simulink model "Nparticles"  (R2025b)
settings: Solver=ode45  StartTime=0.0  StopTime=T  MaxStep=.1  RelTol=1e-5  AbsTol=1e-6
values from neighbouring files (symbols this model uses):
  k = [1, 1, 2, .5]    [bertrand_simulation_Nagents.m]
  q0 = [0; 0; pi/4; 1; 0; pi]    [bertrand_simulation_2agent.m]    (also in bertrand_simulation_Nagents.m = [0, 0, 0,     0, .5, 0,     0, 1, 0,     0, 1.5, 0,     0, 2)
settings Model: Creator=xincheng  LastModifiedBy=xincheng

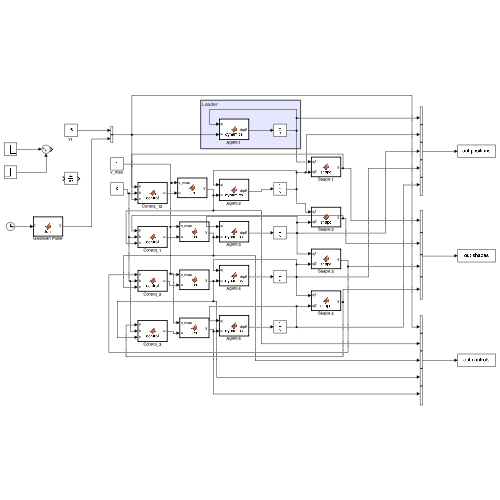
[thumbnail: Simulink's stored preview of the top-level diagram]
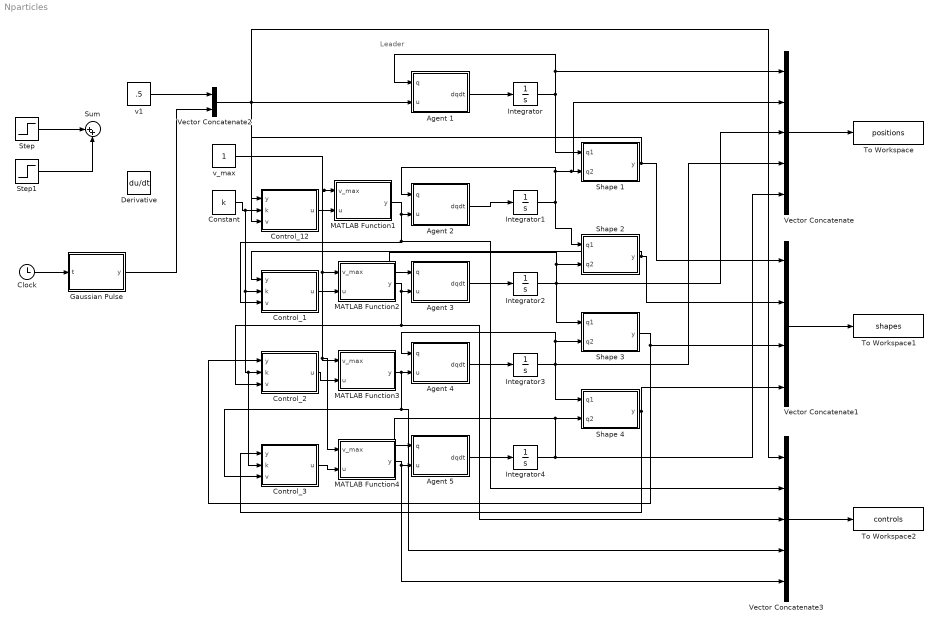
== system Nparticles ==
  note: Leader
  Agent 1 : MATLAB Function  TreatAsAtomicUnit=on
  Agent 2 : MATLAB Function  TreatAsAtomicUnit=on
  Agent 3 : MATLAB Function  TreatAsAtomicUnit=on
  Agent 4 : MATLAB Function  TreatAsAtomicUnit=on
  Agent 5 : MATLAB Function  TreatAsAtomicUnit=on
  Clock : Clock
  Constant : Constant  Value=k
  Control_1 : MATLAB Function  TreatAsAtomicUnit=on
  Control_12 : MATLAB Function  TreatAsAtomicUnit=on
  Control_2 : MATLAB Function  TreatAsAtomicUnit=on
  Control_3 : MATLAB Function  TreatAsAtomicUnit=on
  Derivative : Derivative
  Gaussian Pulse : MATLAB Function  TreatAsAtomicUnit=on
  Integrator : Integrator  InitialCondition=q0(1:3)
  Integrator1 : Integrator  InitialCondition=q0(4:6)
  Integrator2 : Integrator  InitialCondition=q0(7:9)
  Integrator3 : Integrator  InitialCondition=q0(10:12)
  Integrator4 : Integrator  InitialCondition=q0(13:15)
  MATLAB Function1 : MATLAB Function  TreatAsAtomicUnit=on
  MATLAB Function2 : MATLAB Function  TreatAsAtomicUnit=on
  MATLAB Function3 : MATLAB Function  TreatAsAtomicUnit=on
  MATLAB Function4 : MATLAB Function  TreatAsAtomicUnit=on
  Shape 1 : MATLAB Function  TreatAsAtomicUnit=on
  Shape 2 : MATLAB Function  TreatAsAtomicUnit=on
  Shape 3 : MATLAB Function  TreatAsAtomicUnit=on
  Shape 4 : MATLAB Function  TreatAsAtomicUnit=on
  Step : Step  Time=10  After=-2  SampleTime=0
  Step1 : Step  Time=11  After=2  SampleTime=0
  Sum : Sum  Inputs=|++
  To Workspace : ToWorkspace  VariableName=positions  SaveFormat=Timeseries  SampleTime=-1
  To Workspace1 : ToWorkspace  VariableName=shapes  SaveFormat=Timeseries  SampleTime=-1
  To Workspace2 : ToWorkspace  VariableName=controls  SaveFormat=Timeseries  SampleTime=-1
  Vector Concatenate : Concatenate  NumInputs=5
  Vector Concatenate1 : Concatenate  NumInputs=4
  Vector Concatenate2 : Concatenate
  Vector Concatenate3 : Concatenate  NumInputs=5
  v1 : Constant  Value=.5
  v_max : Constant
  wires:
  Agent 1/1(dqdt) -> Integrator/1
  Integrator/1 -> Shape 1/1(q1), Vector Concatenate/1, Agent 1/1(q)
  Integrator1/1 -> Shape 2/1(q1), Agent 2/1(q), Vector Concatenate/2, Shape 1/2(q2)
  Agent 2/1(dqdt) -> Integrator1/1
  Agent 3/1(dqdt) -> Integrator2/1
  Shape 1/1(y) -> Vector Concatenate1/1, Control_12/1(y)
  Control_12/1(u) -> MATLAB Function1/2(u)
  Shape 2/1(y) -> Control_1/1(y), Vector Concatenate1/2
  Control_1/1(u) -> MATLAB Function2/2(u)
  Integrator3/1 -> Shape 4/1(q1), Vector Concatenate/4, Shape 3/2(q2), Agent 4/1(q)
  Shape 3/1(y) -> Control_2/1(y), Vector Concatenate1/3
  Agent 4/1(dqdt) -> Integrator3/1
  Integrator2/1 -> Shape 3/1(q1), Vector Concatenate/3, Shape 2/2(q2), Agent 3/1(q)
  Constant/1 -> Control_1/2(k), Control_3/2(k), Control_2/2(k), Control_12/2(k)
  Control_2/1(u) -> MATLAB Function3/2(u)
  Shape 4/1(y) -> Vector Concatenate1/4, Control_3/1(y)
  Integrator4/1 -> Vector Concatenate/5, Shape 4/2(q2), Agent 5/1(q)
  Control_3/1(u) -> MATLAB Function4/2(u)
  Agent 5/1(dqdt) -> Integrator4/1
  Vector Concatenate/1 -> To Workspace/1
  Vector Concatenate1/1 -> To Workspace1/1
  Vector Concatenate2/1 -> Vector Concatenate3/1, Control_12/3(v), Agent 1/2(u)
  v1/1 -> Vector Concatenate2/1
  Step/1 -> Sum/1
  Step1/1 -> Sum/2
  Vector Concatenate3/1 -> To Workspace2/1
  Clock/1 -> Gaussian Pulse/1(t)
  Gaussian Pulse/1(y) -> Vector Concatenate2/2
  MATLAB Function1/1(y) -> Vector Concatenate3/2, Control_1/3(v), Agent 2/2(u)
  v_max/1 -> MATLAB Function4/1(v_max), MATLAB Function3/1(v_max), MATLAB Function2/1(v_max), MATLAB Function1/1(v_max)
  MATLAB Function2/1(y) -> Vector Concatenate3/3, Control_2/3(v), Agent 3/2(u)
  MATLAB Function3/1(y) -> Control_3/3(v), Vector Concatenate3/4, Agent 4/2(u)
  MATLAB Function4/1(y) -> Vector Concatenate3/5, Agent 5/2(u)

== matlab function Nparticles/Control_3 ==
  data: y input; u output; k input; v input
function u = control(y, k, v)
    u = zeros(1, 2);
    % Unpacking variables
    rho = y(1); alpha1 = y(2); alpha2 = y(3);
    k1 = k(1); k2 = k(2); k_rho = k(3); rho0 = k(4);
    v1 = v(1); u1 = v(2);

    % Calculate and alpha desired
    alpha1_d = pi/2;
    alpha2_d = wrapToPi(alpha1_d + pi); 
    
    f_rho = k_rho * (rho.^2-rho0^2)./rho.^2;

    % Calculate Controls 
    % Lyapunov function V = 1 - cos(alpha1_err) + 1 - cos(alpha2_err)
    %                       + h(rho)
    
    v2 = v1 .* sin(alpha1) - rho .* u1 + rho .* k1 .* sin(alpha1-alpha1_d) + rho .* v1 .* f_rho;
    
    u2 = (v1 .* sin(alpha1) + v2 .* sin(alpha2)) ./ rho + k2 .* sin(alpha2 - alpha2_d);
    u = [v2, u2];
end

== matlab function Nparticles/Agent 2 ==
  data: q input; u input; dqdt output
function dqdt = dynamics(q, u)
    % Unpack states and controls
    x1 = q(1); y1 = q(2); th1 = q(3);
    
    v1 = u(1);
    u1 = u(2);
    % Dynamics
    dqdt = zeros(1,3);

    % Agent dynamics
    dqdt(1) = v1 * cos(th1);
    dqdt(2) = v1 * sin(th1);
    dqdt(3) = u1;
end

== matlab function Nparticles/Shape 4 ==
  data: q1 input; y output; q2 input
function y = shape(q1, q2)
    y = zeros(1, 3);
    % Unpack Global States
    x1 = q1(1); y1 = q1(2); th1 = q1(3);
    x2 = q2(1); y2 = q2(2); th2 = q2(3);
    
    % Calculate Shape Variables
    dx = x2 - x1;
    dy = y2 - y1;
    rho = sqrt(dx^2 + dy^2);
    phi12 = atan2(dy, dx);
    phi21 = atan2(-dy, -dx);

    alpha1 = wrapToPi(phi12 - th1);
    alpha2 = wrapToPi(phi21 - th2);
    
    y = [rho, alpha1, alpha2];
end

== matlab function Nparticles/Gaussian Pulse ==
  data: t input; y output
function y = fcn(t)
    % Define parameters
    a = 1;      % Peak amplitude
    b = 5;      % Time of peak
    c = 1;      % Standard deviation / width

    % Calculate Gaussian pulse
 y = -a * exp(-((t - b)^2) / (2 * c^2));

== matlab function Nparticles/MATLAB Function1 ==
  data: v_max input; u input; y output
function y = fcn(v_max, u)
    v2 = u(1);
    u2 = u(2);
    v = min(v_max, v2);
y = [v u2];

== matlab function Nparticles/MATLAB Function2 ==
  data: v_max input; u input; y output
function y = fcn(v_max, u)
    v2 = u(1);
    u2 = u(2);
    v = min(v_max, v2);
y = [v u2];

== matlab function Nparticles/MATLAB Function3 ==
  data: v_max input; u input; y output
function y = fcn(v_max, u)
    v2 = u(1);
    u2 = u(2);
    v = min(v_max, v2);
y = [v u2];

== matlab function Nparticles/MATLAB Function4 ==
  data: v_max input; u input; y output
function y = fcn(v_max, u)
    v2 = u(1);
    u2 = u(2);
    v = min(v_max, v2);
y = [v u2];

== matlab function Nparticles/Agent 1 ==
  data: q input; u input; dqdt output
function dqdt = dynamics(q, u)
    % Unpack states and controls
    x1 = q(1); y1 = q(2); th1 = q(3);
    
    v1 = u(1);
    u1 = u(2);
    % Dynamics
    dqdt = zeros(1,3);

    % Agent dynamics
    dqdt(1) = v1 * cos(th1);
    dqdt(2) = v1 * sin(th1);
    dqdt(3) = u1;
end

== matlab function Nparticles/Agent 3 ==
  data: q input; u input; dqdt output
function dqdt = dynamics(q, u)
    % Unpack states and controls
    x1 = q(1); y1 = q(2); th1 = q(3);
    
    v1 = u(1);
    u1 = u(2);
    % Dynamics
    dqdt = zeros(1,3);

    % Agent dynamics
    dqdt(1) = v1 * cos(th1);
    dqdt(2) = v1 * sin(th1);
    dqdt(3) = u1;
end

== matlab function Nparticles/Shape 1 ==
  data: q1 input; y output; q2 input
function y = shape(q1, q2)
    y = zeros(1, 3);
    % Unpack Global States
    x1 = q1(1); y1 = q1(2); th1 = q1(3);
    x2 = q2(1); y2 = q2(2); th2 = q2(3);
    
    % Calculate Shape Variables
    dx = x2 - x1;
    dy = y2 - y1;
    rho = sqrt(dx^2 + dy^2);
    phi12 = atan2(dy, dx);
    phi21 = atan2(-dy, -dx);

    alpha1 = wrapToPi(phi12 - th1);
    alpha2 = wrapToPi(phi21 - th2);
    
    y = [rho, alpha1, alpha2];
end

== matlab function Nparticles/Control_12 ==
  data: y input; u output; k input; v input
function u = control(y, k, v)
    u = zeros(1, 2);
    % Unpacking variables
    rho = y(1); alpha1 = y(2); alpha2 = y(3);
    k1 = k(1); k2 = k(2); k_rho = k(3); rho0 = k(4);
    v1 = v(1); u1 = v(2);

    % Calculate and alpha desired
    alpha1_d = pi/2;
    alpha2_d = wrapToPi(alpha1_d + pi); 
    
    f_rho = k_rho * (rho.^2-rho0^2)./rho.^2;

    % Calculate Controls 
    % Lyapunov function V = 1 - cos(alpha1_err) + 1 - cos(alpha2_err)
    %                       + h(rho)
    
    v2 = v1 .* sin(alpha1) - rho .* u1 + rho .* k1 .* sin(alpha1-alpha1_d) + rho .* v1 .* f_rho;
    
    u2 = (v1 .* sin(alpha1) + v2 .* sin(alpha2)) ./ rho + k2 .* sin(alpha2 - alpha2_d);
    u = [v2, u2];
end

== matlab function Nparticles/Shape 2 ==
  data: q1 input; y output; q2 input
function y = shape(q1, q2)
    y = zeros(1, 3);
    % Unpack Global States
    x1 = q1(1); y1 = q1(2); th1 = q1(3);
    x2 = q2(1); y2 = q2(2); th2 = q2(3);
    
    % Calculate Shape Variables
    dx = x2 - x1;
    dy = y2 - y1;
    rho = sqrt(dx^2 + dy^2);
    phi12 = atan2(dy, dx);
    phi21 = atan2(-dy, -dx);

    alpha1 = wrapToPi(phi12 - th1);
    alpha2 = wrapToPi(phi21 - th2);
    
    y = [rho, alpha1, alpha2];
end

== matlab function Nparticles/Control_1 ==
  data: y input; u output; k input; v input
function u = control(y, k, v)
    u = zeros(1, 2);
    % Unpacking variables
    rho = y(1); alpha1 = y(2); alpha2 = y(3);
    k1 = k(1); k2 = k(2); k_rho = k(3); rho0 = k(4);
    v1 = v(1); u1 = v(2);

    % Calculate and alpha desired
    alpha1_d = pi/2;
    alpha2_d = wrapToPi(alpha1_d + pi); 
    
    f_rho = k_rho * (rho.^2-rho0^2)./rho.^2;

    % Calculate Controls 
    % Lyapunov function V = 1 - cos(alpha1_err) + 1 - cos(alpha2_err)
    %                       + h(rho)
    
    v2 = v1 .* sin(alpha1) - rho .* u1 + rho .* k1 .* sin(alpha1-alpha1_d) + rho .* v1 .* f_rho;
    
    u2 = (v1 .* sin(alpha1) + v2 .* sin(alpha2)) ./ rho + k2 .* sin(alpha2 - alpha2_d);
    u = [v2, u2];
end

== matlab function Nparticles/Agent 4 ==
  data: q input; u input; dqdt output
function dqdt = dynamics(q, u)
    % Unpack states and controls
    x1 = q(1); y1 = q(2); th1 = q(3);
    
    v1 = u(1);
    u1 = u(2);
    % Dynamics
    dqdt = zeros(1,3);

    % Agent dynamics
    dqdt(1) = v1 * cos(th1);
    dqdt(2) = v1 * sin(th1);
    dqdt(3) = u1;
end

== matlab function Nparticles/Control_2 ==
  data: y input; u output; k input; v input
function u = control(y, k, v)
    u = zeros(1, 2);
    % Unpacking variables
    rho = y(1); alpha1 = y(2); alpha2 = y(3);
    k1 = k(1); k2 = k(2); k_rho = k(3); rho0 = k(4);
    v1 = v(1); u1 = v(2);

    % Calculate and alpha desired
    alpha1_d = pi/2;
    alpha2_d = wrapToPi(alpha1_d + pi); 
    
    f_rho = k_rho * (rho.^2-rho0^2)./rho.^2;

    % Calculate Controls 
    % Lyapunov function V = 1 - cos(alpha1_err) + 1 - cos(alpha2_err)
    %                       + h(rho)
    
    v2 = v1 .* sin(alpha1) - rho .* u1 + rho .* k1 .* sin(alpha1-alpha1_d) + rho .* v1 .* f_rho;
    
    u2 = (v1 .* sin(alpha1) + v2 .* sin(alpha2)) ./ rho + k2 .* sin(alpha2 - alpha2_d);
    u = [v2, u2];
end

== matlab function Nparticles/Shape 3 ==
  data: q1 input; y output; q2 input
function y = shape(q1, q2)
    y = zeros(1, 3);
    % Unpack Global States
    x1 = q1(1); y1 = q1(2); th1 = q1(3);
    x2 = q2(1); y2 = q2(2); th2 = q2(3);
    
    % Calculate Shape Variables
    dx = x2 - x1;
    dy = y2 - y1;
    rho = sqrt(dx^2 + dy^2);
    phi12 = atan2(dy, dx);
    phi21 = atan2(-dy, -dx);

    alpha1 = wrapToPi(phi12 - th1);
    alpha2 = wrapToPi(phi21 - th2);
    
    y = [rho, alpha1, alpha2];
end

== matlab function Nparticles/Agent 5 ==
  data: q input; u input; dqdt output
function dqdt = dynamics(q, u)
    % Unpack states and controls
    x1 = q(1); y1 = q(2); th1 = q(3);
    
    v1 = u(1);
    u1 = u(2);
    % Dynamics
    dqdt = zeros(1,3);

    % Agent dynamics
    dqdt(1) = v1 * cos(th1);
    dqdt(2) = v1 * sin(th1);
    dqdt(3) = u1;
end
